simulink model "Part1_Peregrin_Falcon_Dive"  (R2022b)
settings: Solver=VariableStepAuto  StartTime=0.0  StopTime=10.0  RelTol=1e-3
undefined symbols (not defined in the file): A, Cd, g, m, rho
settings Model: Creator=Haina Bhawnani  LastModifiedBy=Haina Bhawnani

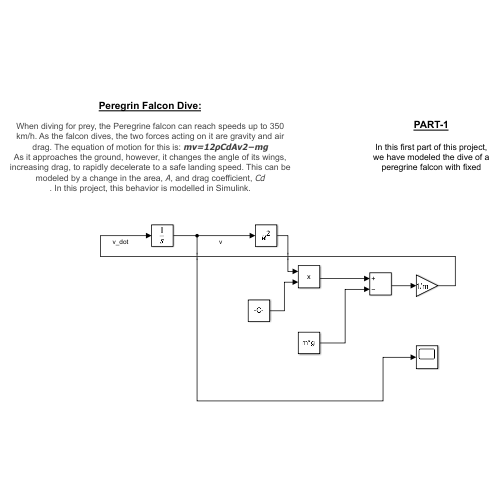
[thumbnail: Simulink's stored preview of the top-level diagram]
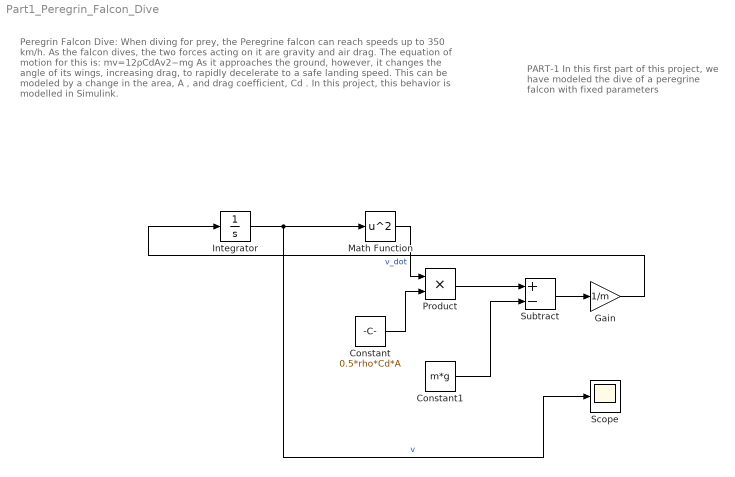
== system Part1_Peregrin_Falcon_Dive ==
  note: Peregrin Falcon Dive:
      |
      | When diving for prey, the Peregrine falcon can reach speeds up to 350 km/h. As the falcon dives, the two forces acting on it are gravity and air drag. The equation of motion for this is: mv=12ρCdAv2−mg
      | As it approaches the ground, however, it changes the angle of its wings, increasing drag, to rapidly decelerate to a safe landing speed. This can be modeled by a change in the area, A , and drag coefficient, Cd
      | . In this project, this behavior is modelled in Simulink.
  note: PART-1
      |
      | In this first part of this project, we have modeled the dive of a peregrine falcon with fixed parameters
  Constant : Constant  Value=0.5*rho*Cd*A
  Constant1 : Constant  Value=m*g
  Gain : Gain  Gain=1/m
  Integrator : Integrator  InitialCondition=-10
  Math Function : Math  Operator=square
  Product : Product
  Scope : Scope
  Subtract : Sum  Inputs=+-
  wires:
  Subtract/1 -> Gain/1
  Product/1 -> Subtract/1
  Constant/1 -> Product/2
  Math Function/1 -> Product/1
  Integrator/1 -> Scope/1, Math Function/1  "v"
  Constant1/1 -> Subtract/2
  Gain/1 -> Integrator/1  "v_dot"
